simulink model "SpeedHarm"  (Simulink 8.2)
settings: Solver=ode1  StartTime=0.0  StopTime=Inf  FixedStep=0.001  RelTol=1e-3
PostLoadFcn:
  | , if any(exist('dsrtsu_mdlpostloadfcn', 'file') == [2, 3, 6]), try dsrtsu_mdlpostloadfcn('Execute', bdroot); catch fprintf('Error in PostLoadFcn (dsrtsu_mdlpostloadfcn) for model "%s":\n %s\n', bdroot, lasterr); end, end,
undefined symbols (not defined in the file): AccelCommandMode, AutoStateEnum, command_mode, max_accel_m_s2, override_enabled, speed_command_m_s, wrench_effort_command
libraries: simulink x33, carma_platform x3, srx_platform x3, dsrc_transmitter x2, rtiethernetudplib x2, rtitttasklib x2, parse_utils x1, rtican x1
(part 1 of 2)
settings Model: DSRTSU_INTERNAL_RTI_VER=450  DSRTSU_INTERNAL_RTI_TYPE=rti1401  DSRTSU_INTERNAL_RTIFPGA=40  Creator=rushk1  LastModifiedBy=leslieem  BufferReuse=off
settings DataIOCC: SignalLoggingSaveFormat=Dataset
settings OptimizationCC: BlockReduction=off  OptimizeBlockIOStorage=off  BufferReuse=off  ExpressionFolding=off  ExpressionDepthLimit=128  LocalBlockOutputs=off
settings DebuggingCC: FcnCallInpInsideContextMsg=EnableAllAsError  StateNameClashWarn=none
settings HardwareCC: ProdIntDivRoundTo=Zero  ProdEndianess=BigEndian  ProdHWDeviceType=Generic->Custom  TargetHWDeviceType=Generic->Custom
settings RTWCC: SystemTargetFile=rti1401.tlc  MakeCommand=make_rti  TemplateMakefile=rti1401.tmf  Description=dSPACE DS1401 Hardware Platform  ProcessScript=rti1401_make_rtw_hook  CustomSource=command_accel_encode.c
settings STFCustomTargetCC: CodeReplacementLibrary=ANSI_C  ParMdlRefBuildCompliant=on  GeneratePreprocessorConditionals=Disable all  SystemTargetFile=rti1401.tlc
settings GRTTargetCC: CompOptLevelCompliant=off  ConcurrentExecutionCompliant=off  MatFileLogging=off  ExtModeMexFile=noextcomm
settings CustomProperty: DataType=RTWOptions_EnumType_C__Program Files_dSPACE RCPHIL 2014-B_MATLAB_RTI_RTI1401_TLC_rti1401_1InitialSimState  Value=RUN
settings EnumStrPairs: String=RUN

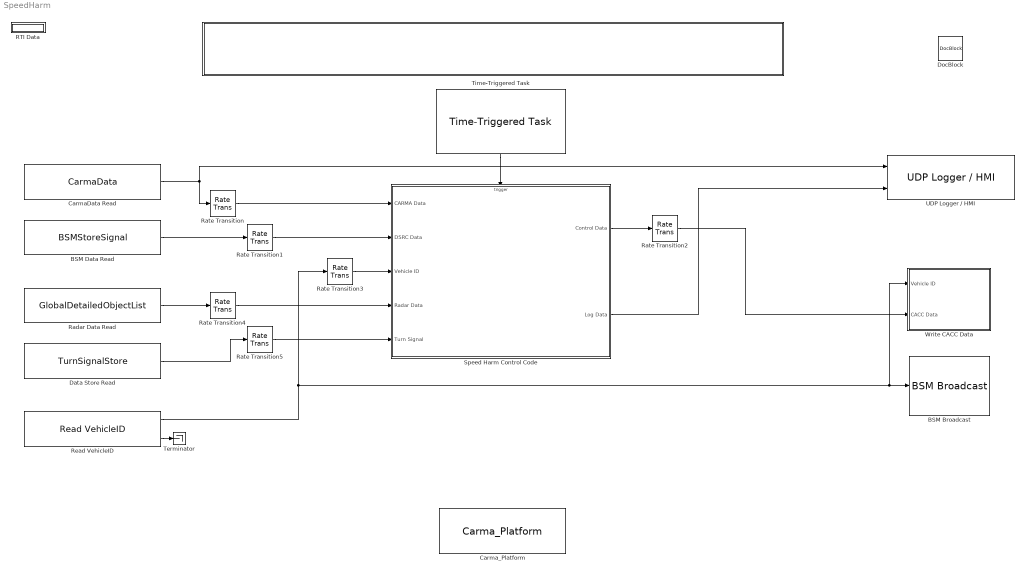
== system SpeedHarm ==
  " " : Subsystem
      mask Display: disp('Speed Harm Control Software\nTOPR 22\n2016')
  BSM Broadcast : dsrc_transmitter/BSM Broadcast
  BSM Data Read : DataStoreRead  DataStoreName=BSMStoreSignal
  CarmaData Read : DataStoreRead  DataStoreName=CarmaData
  "Carma_Platform " : carma_platform/Carma_Platform 
  Data Store Read : DataStoreRead  DataStoreName=TurnSignalStore
  DocBlock : simulink/Model-Wide Utilities/DocBlock  DocumentType=Text
  RTI Data : Subsystem  Tag=struct('RTIDataServer',struct('RTIDataServerVs','2','RTIModelDescription','struct(''main'',''SpeedHarm'',''sub'',''SpeedHarm'',''isMp'',0)'))  LoadFcn="if exist('rtidc'), try,  rtidc('DataHostBlockClbLoad', gcbh); catch, disp(['Warning: ''LoadFcn'' for RTI Data block failed: ' lasterr]); end, end,"  mask(RTI_DATA_HOST){}
      mask help:
      | RTI Data Block.
      | This block is used by RTI to store internal model-dependent data.
      | Please keep this block on the root level of the model. Deleting this block will result in data loss.
      |
      | NEVER DELETE OR COPY THIS BLOCK!
      settings: CopyFcn="if exist('rtidc'), try,  rtidc('DataHostBlockClbCopy', gcbh); catch, disp(['Warning: ''CopyFcn'' for RTI Data block failed: ' lasterr]); end, end,"  DeleteFcn="if exist('rtidc'), try,  rtidc('DataHostBlockClbDelete', gcbh); catch, disp(['Warning: ''DeleteFcn'' for RTI Data block failed: ' lasterr]); end, end,"  ModelCloseFcn="if exist('rtidc'), try,  rtidc('DataHostBlockClbModelClose', gcbh); catch, disp(['Warning: ''ModelCloseFcn'' for RTI Data block failed: ' lasterr]); end, end,"  PreSaveFcn="if exist('rtidc'), try,  rtidc('DataHostBlockClbPreSave', gcbh); catch, disp(['Warning: ''PreSaveFcn'' for RTI Data block failed: ' lasterr]); end, end,"  PostSaveFcn="if exist('rtidc'), try,  rtidc('DataHostBlockClbPostSave', gcbh); catch, disp(['Warning: ''PostSaveFcn'' for RTI Data block failed: ' lasterr]); end, end,"  NameChangeFcn="if exist('rtidc'), try,  rtidc('DataHostBlockClbNameChange', gcbh); catch, disp(['Warning: ''NameChangeFcn'' for RTI Data block failed: ' lasterr]); end, end,"
      mask Help:
      | RTI Data Block.
      | This block is used by RTI to store internal model-dependent data.
      | Please keep this block on the root level of the model. Deleting this block will result in data loss.
      | 
      | NEVER DELETE OR COPY THIS BLOCK!
      mask Display:
      | text(0.5, 0.5, 'RTI Data', 'HorizontalAlignment', 'center');
      | plot([1 0]);
  Radar Data Read : DataStoreRead  DataStoreName=GlobalDetailedObjectList
  Rate Transition{,1..5} (6 alike) : RateTransition  Deterministic=off
  Read VehicleID : srx_platform/Read VehicleID
  Speed Harm Control Code : Subsystem
  Terminator : Terminator
  Time-Triggered Task : rtitttasklib/Time-Triggered Task  TimeTriggerId=ALGO_EXEC  TLCFileName=rtitimetriggeredtask  DSProperties=struct('RTI',struct('Version',uint32(1),'BlockType',struct('isSLSource',uint8(1),'isSLSink',uint8(0),'isHWSource',uint8(0),'isHWSink',uint8(0),'isSetup',uint8(0),'isInline',uint8(1),'isNonInline',uint8(0),'isInterrupt',uint8(0),'isChannelwise',uint8(0)),'IOBoardType','RTITIMETRIGGER','UnitType','TIMETRIGGERED','Identifier','TASK','DialogType','SL','BlockSet','NONE','SlaveProcessor','NONE'))  RTIBlockInterface=struct('OutputPortsActive',1,'OutputPortsWidth',int32(1),'FunctionCall',uint32(0),'OutputPortsName',{{[' ']}},'InitLevel',3,'BlockDisplay',{{['Time-Triggered Task\nID: ''''ALGO_EXEC'''''],'center'}},'IconTransparency','off','BlockName',struct('Token',{{['Time-Triggered Task']}}),'MaskDescription',['Specifies a time-triggered task. The task trigger times are set by the assigned Time-Trigger Set block.' char(10) '' char(10) 'This block can only be used together with the Time-Trigger Set block.'])  RTIBlockParameters=struct('TimeTriggerId',{{'ALGO_EXEC','OFF',[]}},'TLCFileName',{{'rtitimetriggeredtask','OFF',[]}})  RTISFcnParameters=struct('TLCFileName','char')  RTIBlockParaDefault=struct('TimeTriggerId','TT_ID','TLCFileName','rtitimetriggeredtask')
  UDP Logger / HMI : carma_platform/UDP Logger // HMI  Value=0.05
  Write CACC Data : Subsystem  AncestorBlock=dsrc_transmitter/Write CACC Data
  wires:
  BSM Data Read/1 -> Rate Transition1/1
  CarmaData Read/1 -> Rate Transition/1, UDP Logger / HMI/1
  Rate Transition1/1 -> Speed Harm Control Code/2(DSRC Data)
  Speed Harm Control Code/2(Log Data) -> UDP Logger / HMI/2
  Speed Harm Control Code/1(Control Data) -> Rate Transition2/1
  Read VehicleID/2 -> Terminator/1
  Read VehicleID/1 -> Write CACC Data/1(Vehicle ID), BSM Broadcast/1, Rate Transition3/1
  Rate Transition2/1 -> Write CACC Data/2(CACC Data)
  Time-Triggered Task/1 -> Speed Harm Control Code/Trigger
  Rate Transition3/1 -> Speed Harm Control Code/3(Vehicle ID)
  Rate Transition/1 -> Speed Harm Control Code/1(CARMA Data)
  Radar Data Read/1 -> Rate Transition4/1
  Rate Transition4/1 -> Speed Harm Control Code/4(Radar Data)
  Data Store Read/1 -> Rate Transition5/1
  Rate Transition5/1 -> Speed Harm Control Code/5(Turn Signal)

== system SpeedHarm/  ==

== system SpeedHarm/RTI Data ==
  RTI Data Store : Subsystem  Tag=struct('private',struct('version',struct('dsVer',uint32(2)),'access',struct('modified',['03-May-2016 18:00:07'],'type','Model','isPerm',1)))  mask(RTI_DATA_STORE){}
      mask help:
      | RTI Data Store Block. This block is used by RTI to store internal model dependent data. Deleting this block will result in data loss.
      |
      | NEVER DELETE, COPY, OR MODIFY THIS BLOCK!
      mask Help:
      | RTI Data Store Block. This block is used by RTI to store internal model dependent data. Deleting this block will result in data loss.
      | 
      | NEVER DELETE, COPY, OR MODIFY THIS BLOCK!
      mask Display: text(0.5, 0.5, ' ', 'HorizontalAlignment', 'center');

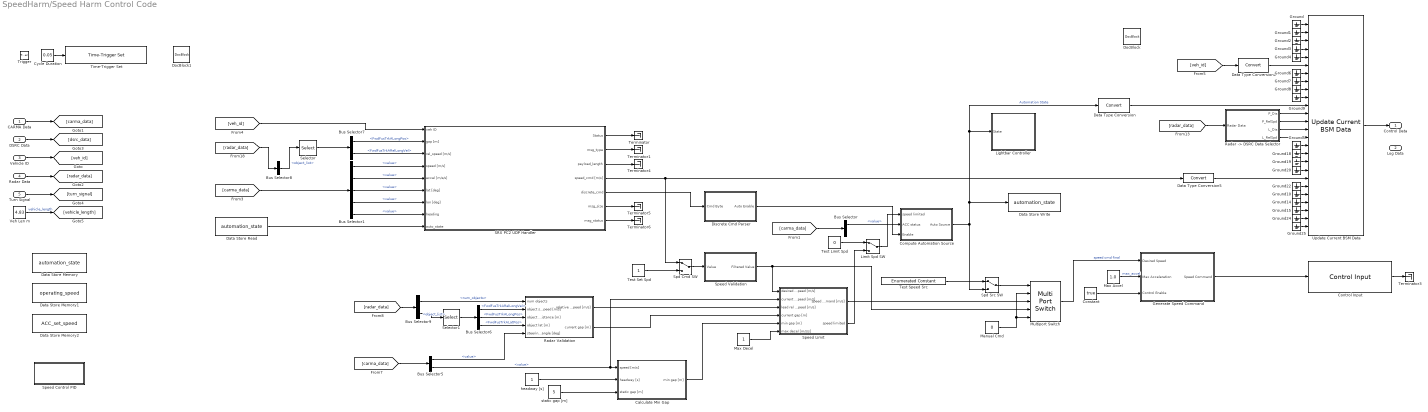
== system SpeedHarm/Speed Harm Control Code ==
  CARMA Data : Inport
  DSRC Data : Inport  Port=2
  Vehicle ID : Inport  Port=3
  Radar Data : Inport  Port=4  OutDataTypeStr=Bus: DetailedObjectList
  Turn Signal : Inport  Port=5
  Trigger : TriggerPort  TriggerType=function-call  PortDimensions=1
  Bus Selector : BusSelector  OutputSignals=acc_status.value,requested_cacc_state.value
  Bus Selector1 : BusSelector  OutputSignals=speed_m_s.value,accel_m_s2.value,global_lat_deg.value,global_long_deg.value,global_yaw_deg.value
  Bus Selector5 : BusSelector  OutputSignals=steering_wheel_angle_deg.value,speed_m_s.value
  Bus Selector6 : BusSelector  OutputSignals=FwdFusTrkARelLongVel,FwdFusTrkALongPos,FwdFusTrkALatPos
  Bus Selector7 : BusSelector  OutputSignals=FwdFusTrkALongPos,FwdFusTrkARelLongVel
  Bus Selector8 : BusSelector  OutputSignals=object_list
  Bus Selector9 : BusSelector  OutputSignals=num_objects,object_list
  Calculate Min Gap : Subsystem
  Compute Automation Source : Subsystem
  Constant : Constant  Value=true
  Control Input : carma_platform/Control Input
  Cycle Duration : Constant  Value=0.05
  Data Store Memory : DataStoreMemory  DataStoreName=automation_state  ReadBeforeWriteMsg=warning  WriteAfterWriteMsg=warning  WriteAfterReadMsg=warning  InitialValue=AutoStateEnum.MANUAL  OutDataTypeStr=Enum: AutoStateEnum
  Data Store Memory1 : DataStoreMemory  DataStoreName=operating_speed  ReadBeforeWriteMsg=warning  WriteAfterWriteMsg=warning  WriteAfterReadMsg=warning  InitialValue=25
  Data Store Memory2 : DataStoreMemory  DataStoreName=ACC_set_speed  ReadBeforeWriteMsg=warning  WriteAfterWriteMsg=warning  WriteAfterReadMsg=warning  InitialValue=25
  Data Store Read : DataStoreRead  DataStoreName=automation_state  DataStoreElements=automation_state
  Data Store Write : DataStoreWrite  DataStoreName=automation_state  DataStoreElements=automation_state
  Data Type Conversion : DataTypeConversion
  Data Type Conversion1 : DataTypeConversion
  Data Type Conversion5 : DataTypeConversion
  Discrete Cmd Parser : Subsystem
  DocBlock : simulink/Model-Wide Utilities/DocBlock  DocumentType=Text
  DocBlock1 : simulink/Model-Wide Utilities/DocBlock  DocumentType=Text
      content=|
      | Speed Harmonization Control Code
      | ===========================================================================
      | This subystem contains all of the algorithm logic for the Speed
      | Harmonization (Speed Harm) application.
      |
      | This logic is executed at a 20hz timestep with hard real time deadlines.
      | During each iteration the following steps are performed:
      |
      | 1) Receive inputs from the platform. The latest data are gathered from the
      | relevant storage buffers (being updated by other code on independent time
      | basis) and used to perform new computations.
      | 2) Receive speed command from Secondary PC
      | 3) Package vehicle data to send to Secondary PC
      | 4) Broadcast data. The new state, speed command, and other data is written
      | into the appropriate DSRC buffers and broadcasted.
  Generate Speed Command : Subsystem
  Ground{,1..10,14..15,18..20,22,24..25} (19 alike) : Ground
  Lightbar Controller : Subsystem
  Limit Spd SW : ManualSwitch
  Manual Cmd : Constant  Value=0
  Max Accel : Constant  Value=1.0
  Max Decel : Constant
  Multiport Switch : MultiPortSwitch  DataPortOrder=Specify indices  DataPortIndices={AutoStateEnum.MANUAL, AutoStateEnum.AUTO_LOCAL, AutoStateEnum.AUTO_FULL}  DataPortForDefault=Additional data port
  "Radar -> DSRC Data Selector" : Subsystem
  Radar Validation : Subsystem
  SRX PC2 UDP Handler : Subsystem
  Selector : Selector  IndexMode=Zero-based  InputPortWidth=4  IndexOptions=Index vector (dialog)  Indices=[0]  OutputSizes=1
  Selector1 : Selector  IndexMode=Zero-based  InputPortWidth=4  IndexOptions=Index vector (dialog)  Indices=[0]  OutputSizes=1
  Spd Cmd SW : ManualSwitch
  Spd Src SW : ManualSwitch
  Speed Control PID : Subsystem
  Speed Limit : Subsystem
  Speed Validation : Subsystem
  Terminator{,1,3..6} (6 alike) : Terminator
  Test Limit Spd : Constant  Value=0
  Test Set Spd : Constant
  Test Speed Src : simulink/Sources/Enumerated Constant  OutDataTypeStr=Enum: AutoStateEnum  Value=AutoStateEnum.AUTO_FULL  SampleTime=inf
  Time-Trigger Set : rtitttasklib/Time-Trigger Set  TimeTriggerId=ALGO_EXEC  SampleTime=-1  RegisterAtSimulationStart=on  TLCFileName=rtitimetriggerset  DSProperties=struct('RTI',struct('Version',uint32(1),'BlockType',struct('isSLSource',uint8(1),'isSLSink',uint8(0),'isHWSource',uint8(0),'isHWSink',uint8(0),'isSetup',uint8(0),'isInline',uint8(1),'isNonInline',uint8(0),'isInterrupt',uint8(0),'isChannelwise',uint8(0)),'IOBoardType','RTITIMETRIGGER','UnitType','TIMETRIGGERED','Identifier','SET','DialogType','SL','BlockSet','NONE','SlaveProcessor','NONE'))  RTIBlockInterface=struct('InputPortsActive',1,'InputPortsWidth',{{'DYNAMICALLY_SIZED'}},'InputPortsDataType',{{'SS_DOUBLE'}},'InputPortsName',{{['Trigger delay']}},'InitLevel',3,'BlockDisplay',{{['Time-Trigger Set\nID: ''''ALGO_EXEC'''''],'center'}},'IconTransparency','on','BlockName',struct('Token',{{['Time-Trigger Set']}}),'MaskDescription',['When this block is evaluated it sets the task trigger times for the assigned time-triggered task.' char(10) '' char(10) 'This block can only be used together with the Time-Triggered Task block.'],'SampleTime',{{-1}})  RTIBlockParameters=struct('TimeTriggerId',{{'ALGO_EXEC','OFF',[]}},'SampleTime',{{-1,'OFF',[]}},'RegisterAtSimulationStart',{{logical(1),'OFF',[]}},'TLCFileName',{{'rtitimetriggerset','OFF',[]}})  RTISFcnParameters=struct('TimeTriggerId','char','SampleTime','double','TLCFileName','char','RegisterAtSimulationStart','double')  RTIBlockParaDefault=struct('TimeTriggerId','TT_ID','SampleTime',-1,'RegisterAtSimulationStart',0,'TLCFileName','rtitimetriggerset')
  Update Current BSM Data : dsrc_transmitter/Update Current BSM Data
  Veh Len m : Constant  Value=4.83
  headway [s] : Constant
  static gap [m] : Constant  Value=5
  Control Data : Outport
  Log Data : Outport  Port=2
  wires:
  Vehicle ID/1 -> [veh_id]
  Cycle Duration/1 -> Time-Trigger Set/1
  Update Current BSM Data/1 -> Control Data/1
  Ground/1 -> Update Current BSM Data/1
  Ground1/1 -> Update Current BSM Data/2
  Ground2/1 -> Update Current BSM Data/3
  Ground3/1 -> Update Current BSM Data/4
  Ground4/1 -> Update Current BSM Data/5
  Ground9/1 -> Update Current BSM Data/10
  Ground7/1 -> Update Current BSM Data/8
  Ground8/1 -> Update Current BSM Data/9
  Ground6/1 -> Update Current BSM Data/7
  Ground22/1 -> Update Current BSM Data/21
  Ground15/1 -> Update Current BSM Data/24
  Ground19/1 -> Update Current BSM Data/18
  Ground18/1 -> Update Current BSM Data/17
  Ground14/1 -> Update Current BSM Data/23
  Ground20/1 -> Update Current BSM Data/19
  Ground24/1 -> Update Current BSM Data/25
  Ground25/1 -> Update Current BSM Data/26
  Radar Data/1 -> [radar_data]
  CARMA Data/1 -> [carma_data]
  Compute Automation Source/1(Auto Source) -> Data Type Conversion/1, Lightbar Controller/1(State), Data Store Write/1, Spd Src SW/2  "Automation State"
  Data Type Conversion1/1 -> Update Current BSM Data/6
  [carma_data] -> Bus Selector/1
  DSRC Data/1 -> [dsrc_data]
  [veh_id] -> Data Type Conversion1/1
  Ground10/1 -> Update Current BSM Data/22
  SRX PC2 UDP Handler/1(Status) -> Terminator/1
  Control Input/1 -> Terminator3/1
  Speed Validation/1(Filtered Value) -> Multiport Switch/4, Speed Limit/1(desired speed [m/s])
  Generate Speed Command/1(Speed Command) -> Control Input/1
  Max Accel/1 -> Generate Speed Command/2(Max Acceleration)  "max_accel"
  Turn Signal/1 -> [turn_signal]
  Ground5/1 -> Update Current BSM Data/16
  [radar_data] -> "Radar -> DSRC Data Selector"/1(Radar Data)
  "Radar -> DSRC Data Selector"/1(P_Dis) -> Update Current BSM Data/12
  "Radar -> DSRC Data Selector"/2(P_RelSpd) -> Update Current BSM Data/13
  "Radar -> DSRC Data Selector"/3(L_Dis) -> Update Current BSM Data/14
  "Radar -> DSRC Data Selector"/4(L_RelSpd) -> Update Current BSM Data/15
  Data Type Conversion5/1 -> Update Current BSM Data/20
  Veh Len m/1 -> [vehicle_length]  "vehicle_length"
  static gap [m]/1 -> Calculate Min Gap/3(static gap [m])
  SRX PC2 UDP Handler/6(msg_size) -> Terminator5/1
  Bus Selector7/1 -> SRX PC2 UDP Handler/2(gap [m])  "<FwdFusTrkALongPos>"
  [carma_data] -> Bus Selector1/1
  Bus Selector1/1 -> SRX PC2 UDP Handler/4(speed [m/s])  "<value>"
  Bus Selector1/2 -> SRX PC2 UDP Handler/5(accel [m/s/s])  "<value>"
  Bus Selector1/3 -> SRX PC2 UDP Handler/6(lat [deg])  "<value>"
  Bus Selector1/4 -> SRX PC2 UDP Handler/7(lon [deg])  "<value>"
  SRX PC2 UDP Handler/7(msg_status) -> Terminator6/1
  SRX PC2 UDP Handler/3(payload_length) -> Terminator4/1
  SRX PC2 UDP Handler/2(msg_type) -> Terminator1/1
  [veh_id] -> SRX PC2 UDP Handler/1(veh ID)
  Bus Selector1/5 -> SRX PC2 UDP Handler/8(heading)  "<value>"
  Bus Selector7/2 -> SRX PC2 UDP Handler/3(rel_speed [m/s])  "<FwdFusTrkARelLongVel>"
  SRX PC2 UDP Handler/4(speed_cmd [m/s]) -> Spd Cmd SW/1, Data Type Conversion5/1
  Constant/1 -> Generate Speed Command/3(Control Enable)
  headway [s]/1 -> Calculate Min Gap/2(headway [s])
  [carma_data] -> Bus Selector5/1
  Bus Selector5/2 -> Speed Limit/2(current speed [m/s]), Calculate Min Gap/1(speed [m/s])  "<value>"
  Bus Selector6/2 -> Radar Validation/3(object distance [m])  "<FwdFusTrkALongPos>"
  Calculate Min Gap/1(min gap [m]) -> Speed Limit/5(min gap [m])
  Radar Validation/2(current gap [m]) -> Speed Limit/4(current gap [m])
  Bus Selector9/1 -> Radar Validation/1(num objects)  "<num_objects>"
  Radar Validation/1(relative speed [m/s]) -> Speed Limit/3(lead rel speed [m/s])
  Bus Selector6/1 -> Radar Validation/2(object speed [m/s])  "<FwdFusTrkARelLongVel>"
  Speed Limit/1(speed command [m/s]) -> Multiport Switch/3
  [radar_data] -> Bus Selector8/1
  Bus Selector8/1 -> Selector/1  "<object_list>"
  Selector/1 -> Bus Selector7/1
  Selector1/1 -> Bus Selector6/1
  Bus Selector9/2 -> Selector1/1  "<object_list>"
  Data Type Conversion/1 -> Update Current BSM Data/11
  SRX PC2 UDP Handler/5(discrete_cmd) -> Discrete Cmd Parser/1(Cmd Byte)
  Data Store Read/1 -> SRX PC2 UDP Handler/9(auto_state)
  Manual Cmd/1 -> Multiport Switch/5, Multiport Switch/2
  [radar_data] -> Bus Selector9/1
  Discrete Cmd Parser/1(Auto Enable) -> Compute Automation Source/3(Enable)
  Limit Spd SW/1 -> Compute Automation Source/1(speed limited)
  Test Set Spd/1 -> Spd Cmd SW/2
  Spd Cmd SW/1 -> Speed Validation/1(Value)
  Multiport Switch/1 -> Generate Speed Command/1(Desired Speed)  "speed cmd final"
  Test Speed Src/1 -> Spd Src SW/1
  Spd Src SW/1 -> Multiport Switch/1
  Bus Selector/1 -> Compute Automation Source/2(ACC status)  "<value>"
  Test Limit Spd/1 -> Limit Spd SW/1
  Max Decel/1 -> Speed Limit/6(max decel [m/s/s])
  Speed Limit/2(speed limited) -> Limit Spd SW/2
  Bus Selector5/1 -> Radar Validation/5(steering angle [deg])  "<value>"
  Bus Selector6/3 -> Radar Validation/4(object lat [m])  "<FwdFusTrkALatPos>"

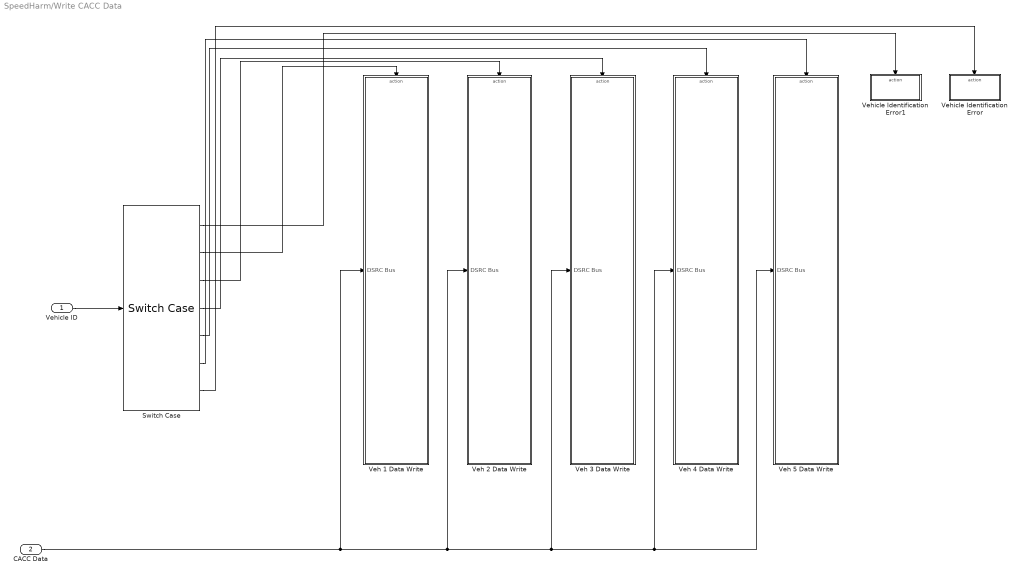
== system SpeedHarm/Write CACC Data ==
  Vehicle ID : Inport
  CACC Data : Inport  Port=2
  Switch Case : SwitchCase  CaseConditions={0,96,97,98,99,100}
  Veh 1 Data Write : Subsystem  TreatAsAtomicUnit=on
  Veh 2 Data Write : Subsystem  TreatAsAtomicUnit=on
  Veh 3 Data Write : Subsystem  TreatAsAtomicUnit=on
  Veh 4 Data Write : Subsystem  TreatAsAtomicUnit=on
  Veh 5 Data Write : Subsystem  TreatAsAtomicUnit=on
  Vehicle Identification Error : Subsystem  TreatAsAtomicUnit=on
  Vehicle Identification Error1 : Subsystem  TreatAsAtomicUnit=on
  wires:
  Vehicle ID/1 -> Switch Case/1
  Switch Case/7 -> Vehicle Identification Error/Action
  Switch Case/1 -> Vehicle Identification Error1/Action
  Switch Case/6 -> Veh 5 Data Write/Action
  Switch Case/5 -> Veh 4 Data Write/Action
  Switch Case/4 -> Veh 3 Data Write/Action
  Switch Case/3 -> Veh 2 Data Write/Action
  Switch Case/2 -> Veh 1 Data Write/Action
  CACC Data/1 -> Veh 1 Data Write/1(DSRC Bus), Veh 2 Data Write/1(DSRC Bus), Veh 3 Data Write/1(DSRC Bus), Veh 4 Data Write/1(DSRC Bus), Veh 5 Data Write/1(DSRC Bus)

== system SpeedHarm/RTI Data/RTI Data Store ==
  RTI Data Store : Subsystem  mask(RTI_DATA_STORE){}
      mask help:
      | RTI Data Store Block. This block is used by RTI to store internal model dependent data. Deleting this block will result in data loss.
      |
      | NEVER DELETE, COPY, OR MODIFY THIS BLOCK!
      mask Help:
      | RTI Data Store Block. This block is used by RTI to store internal model dependent data. Deleting this block will result in data loss.
      | 
      | NEVER DELETE, COPY, OR MODIFY THIS BLOCK!
      mask Display: text(0.5, 0.5, ' ', 'HorizontalAlignment', 'center');

== system SpeedHarm/Speed Harm Control Code/Calculate Min Gap ==
  speed [m/s] : Inport
  headway [s] : Inport  Port=2
  static gap [m] : Inport  Port=3
  Add : Sum
  DocBlock : simulink/Model-Wide Utilities/DocBlock  DocumentType=Text
  Product : Product
  min gap [m] : Outport
  wires:
  static gap [m]/1 -> Add/2
  speed [m/s]/1 -> Product/1
  headway [s]/1 -> Product/2
  Product/1 -> Add/1
  Add/1 -> min gap [m]/1

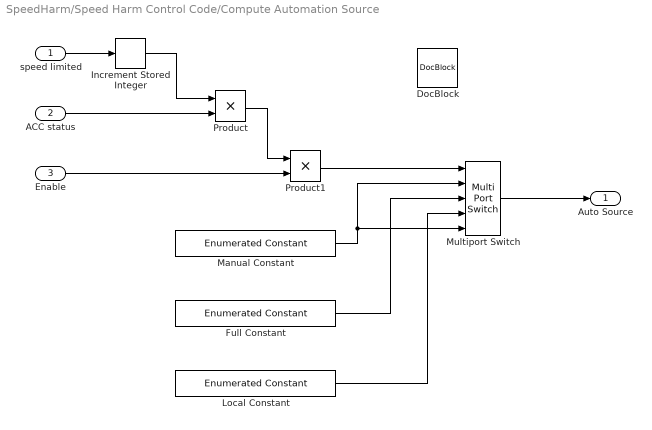
== system SpeedHarm/Speed Harm Control Code/Compute Automation Source ==
  speed limited : Inport
  ACC status : Inport  Port=2
  Enable : Inport  Port=3
  DocBlock : simulink/Model-Wide Utilities/DocBlock  DocumentType=Text
  Full Constant : simulink/Sources/Enumerated Constant  OutDataTypeStr=Enum: AutoStateEnum  Value=AutoStateEnum.AUTO_FULL  SampleTime=inf
  Increment Stored Integer : simulink/Additional Math & Discrete/Additional Math: Increment - Decrement/Increment Stored Integer
  Local Constant : simulink/Sources/Enumerated Constant  OutDataTypeStr=Enum: AutoStateEnum  Value=AutoStateEnum.AUTO_LOCAL  SampleTime=inf
  Manual Constant : simulink/Sources/Enumerated Constant  OutDataTypeStr=Enum: AutoStateEnum  Value=AutoStateEnum.MANUAL  SampleTime=inf
  Multiport Switch : MultiPortSwitch  DataPortOrder=Zero-based contiguous  DataPortForDefault=Additional data port
  Product : Product
  Product1 : Product
  Auto Source : Outport
  wires:
  Multiport Switch/1 -> Auto Source/1
  Manual Constant/1 -> Multiport Switch/5, Multiport Switch/2
  Full Constant/1 -> Multiport Switch/3
  Local Constant/1 -> Multiport Switch/4
  Product1/1 -> Multiport Switch/1
  ACC status/1 -> Product/2
  speed limited/1 -> Increment Stored Integer/1
  Increment Stored Integer/1 -> Product/1
  Product/1 -> Product1/1
  Enable/1 -> Product1/2

== system SpeedHarm/Speed Harm Control Code/Discrete Cmd Parser ==
  Cmd Byte : Inport
  Bitwise Operator : simulink/Logic and Bit Operations/Bitwise Operator  logicop=AND  UseBitMask=on  BitMask=bin2dec('00000001')  BitMaskRealWorld=Stored Integer
  DocBlock : simulink/Model-Wide Utilities/DocBlock  DocumentType=Text
  Auto Enable : Outport
  wires:
  Cmd Byte/1 -> Bitwise Operator/1
  Bitwise Operator/1 -> Auto Enable/1

== system SpeedHarm/Speed Harm Control Code/Generate Speed Command ==
  Desired Speed : Inport
  Max Acceleration : Inport  Port=2
  Control Enable : Inport  Port=3
  Accel Zero Command : Constant  Value=0  OutDataTypeStr=Bus: AccelCommandBus
  Bus Assignment : BusAssignment  AssignedSignals=override_enabled,command_mode,wrench_effort_command,speed_command_m_s,max_accel_m_s2
  Constant : Constant  Value=AccelCommandMode.SpeedControl  OutDataTypeStr=Enum: AccelCommandMode
  Constant1 : Constant  Value=0
  DocBlock : simulink/Model-Wide Utilities/DocBlock  DocumentType=Text
  Speed Command : Outport
  wires:
  Control Enable/1 -> Bus Assignment/2
  Constant1/1 -> Bus Assignment/4
  Desired Speed/1 -> Bus Assignment/5
  Max Acceleration/1 -> Bus Assignment/6
  Accel Zero Command/1 -> Bus Assignment/1
  Bus Assignment/1 -> Speed Command/1
  Constant/1 -> Bus Assignment/3

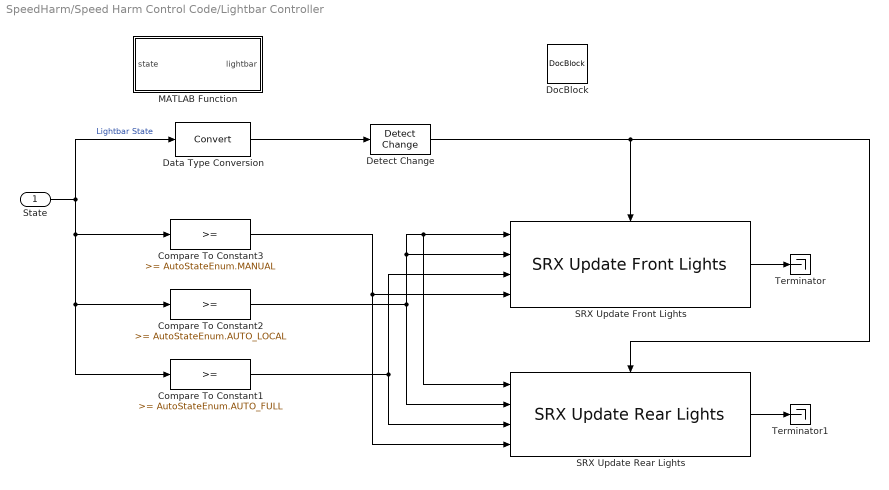
== system SpeedHarm/Speed Harm Control Code/Lightbar Controller ==
  State : Inport
  Compare To Constant1 : simulink/Logic and Bit Operations/Compare To Constant  relop=>=  const=AutoStateEnum.AUTO_FULL  OutDataTypeStr=boolean
  Compare To Constant2 : simulink/Logic and Bit Operations/Compare To Constant  relop=>=  const=AutoStateEnum.AUTO_LOCAL  OutDataTypeStr=boolean
  Compare To Constant3 : simulink/Logic and Bit Operations/Compare To Constant  relop=>=  const=AutoStateEnum.MANUAL  OutDataTypeStr=boolean
  Data Type Conversion : DataTypeConversion
  Detect Change : simulink/Logic and Bit Operations/Detect Change  vinit=0  InputProcessing=Inherited  OutDataTypeStr=boolean
  DocBlock : simulink/Model-Wide Utilities/DocBlock  DocumentType=Text
      content=|
      | This block is responsible for controlling the state of the vehicle's
      | lightbar.
      |
      | The lightbar state is dependant on the vehicle's merge state. Merge request
      | triggers the right side of the lightbar to flash. Merge request ack
      | triggers the left side of the bar to flash. Merge ready causes both sides
      | of the lightbar to flash. Once merge completion is attained the green light
      | in the center of light bar will light up solid.
  MATLAB Function : MATLAB Function  TreatAsAtomicUnit=on
  SRX Update Front Lights : srx_platform/SRX Update Front Lights
  SRX Update Rear Lights : srx_platform/SRX Update Rear Lights
  Terminator : Terminator
  Terminator1 : Terminator
  wires:
  Compare To Constant2/1 -> SRX Update Rear Lights/1, SRX Update Front Lights/1, SRX Update Front Lights/2, SRX Update Rear Lights/2
  Compare To Constant1/1 -> SRX Update Front Lights/3, SRX Update Rear Lights/3
  Compare To Constant3/1 -> SRX Update Rear Lights/4, SRX Update Front Lights/4
  Detect Change/1 -> SRX Update Front Lights/Enable, SRX Update Rear Lights/Enable
  SRX Update Front Lights/1 -> Terminator/1
  SRX Update Rear Lights/1 -> Terminator1/1
  State/1 -> Compare To Constant2/1, Compare To Constant1/1, Compare To Constant3/1, Data Type Conversion/1  "Lightbar State"
  Data Type Conversion/1 -> Detect Change/1

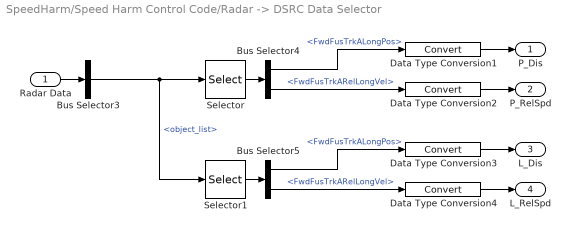
== system SpeedHarm/Speed Harm Control Code/Radar -> DSRC Data Selector ==
  Radar Data : Inport
  Bus Selector3 : BusSelector  OutputSignals=object_list
  Bus Selector4 : BusSelector  OutputSignals=FwdFusTrkALongPos,FwdFusTrkARelLongVel
  Bus Selector5 : BusSelector  OutputSignals=FwdFusTrkALongPos,FwdFusTrkARelLongVel
  Data Type Conversion{1..4} (4 alike) : DataTypeConversion
  Selector : Selector  InputPortWidth=4  IndexOptions=Index vector (dialog)  Indices=[1]  OutputSizes=1
  Selector1 : Selector  InputPortWidth=4  IndexOptions=Index vector (dialog)  Indices=[2]  OutputSizes=1
  P_Dis : Outport
  P_RelSpd : Outport  Port=2
  L_Dis : Outport  Port=3
  L_RelSpd : Outport  Port=4
  wires:
  Bus Selector5/2 -> Data Type Conversion4/1  "<FwdFusTrkARelLongVel>"
  Bus Selector5/1 -> Data Type Conversion3/1  "<FwdFusTrkALongPos>"
  Radar Data/1 -> Bus Selector3/1
  Bus Selector4/2 -> Data Type Conversion2/1  "<FwdFusTrkARelLongVel>"
  Bus Selector3/1 -> Selector1/1, Selector/1  "<object_list>"
  Bus Selector4/1 -> Data Type Conversion1/1  "<FwdFusTrkALongPos>"
  Selector1/1 -> Bus Selector5/1
  Selector/1 -> Bus Selector4/1
  Data Type Conversion1/1 -> P_Dis/1
  Data Type Conversion2/1 -> P_RelSpd/1
  Data Type Conversion3/1 -> L_Dis/1
  Data Type Conversion4/1 -> L_RelSpd/1

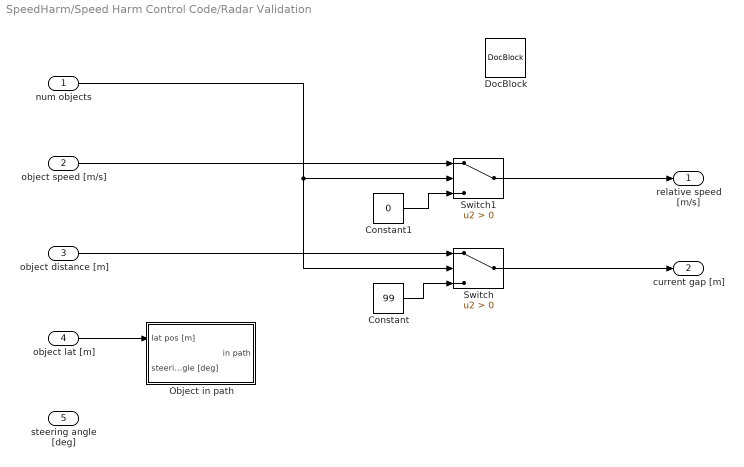
== system SpeedHarm/Speed Harm Control Code/Radar Validation ==
  num objects : Inport
  object speed [m/s] : Inport  Port=2
  object distance [m] : Inport  Port=3
  object lat [m] : Inport  Port=4
  steering angle [deg] : Inport  Port=5
  Constant : Constant  Value=99
  Constant1 : Constant  Value=0
  DocBlock : simulink/Model-Wide Utilities/DocBlock  DocumentType=Text
      content=|
      | This block outputs the radar distance and speed to the nearest object,
      | or outputs a known value if no objects are detected.
      |
      | Future work:
      | Use the radar azimuth, steering wheel angle, and other data to filter out
      | objects not in the path of this vehicle
  Object in path : Subsystem
  Switch : Switch  Criteria=u2 > Threshold
  Switch1 : Switch  Criteria=u2 > Threshold
  relative speed [m/s] : Outport
  current gap [m] : Outport  Port=2
  wires:
  num objects/1 -> Switch/2, Switch1/2
  object distance [m]/1 -> Switch/1
  Constant/1 -> Switch/3
  Switch/1 -> current gap [m]/1
  object speed [m/s]/1 -> Switch1/1
  Constant1/1 -> Switch1/3
  Switch1/1 -> relative speed [m/s]/1
  object lat [m]/1 -> Object in path/1(lat pos [m])

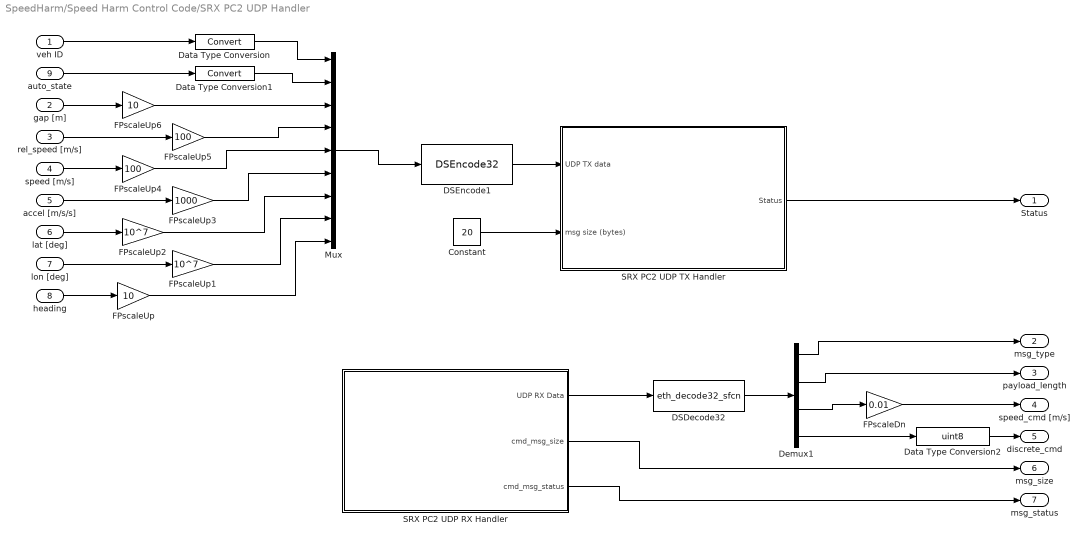
== system SpeedHarm/Speed Harm Control Code/SRX PC2 UDP Handler ==
  veh ID : Inport
  gap [m] : Inport  Port=2
  rel_speed [m/s] : Inport  Port=3
  speed [m/s] : Inport  Port=4
  accel [m/s/s] : Inport  Port=5
  lat [deg] : Inport  Port=6
  lon [deg] : Inport  Port=7
  heading : Inport  Port=8
  auto_state : Inport  Port=9
  Constant : Constant  Value=20  OutDataTypeStr=int32
  "DSDecode32 " : S-Function  FunctionName=eth_decode32_sfcn  Parameters=byteordering,offset,auto_offset,datatype,one_datatype,sampletime  EnableBusSupport=off  mask(DSDecode32){byteordering=little endian (Intel), offset=[0], auto_offset=on, datatype=[3 3 5 3], one_datatype=off, sampletime=-1}
      mask prompts: byteordering "Byte ordering:"; offset "Offset (bytes):"; auto_offset "Auto offset"; one_datatype "One datatype only"
      mask help:
      | Converts a 32bit WORD input data stream into the specified datatypes on the output port.
      |
      | Datatype Codes:
      | BOOLEAN:  1   //   INT8      :  2    //   UINT8    :  3
      | INT16       :  4   //   UINT16 :  5    //   INT32     :  6
      | UINT32    :  7   //   FLOAT   :  8    //   DOUBLE:  9
      mask Help:
      | The 'DSDecode32' block allows to decode an UInt32 vector containing encoded elements of various data types to an output vector of double values. It is intended to use this block in conjunction with the 'DS4504_ETH_Receive' block which delivers this format as data output. Data received from the Ethernet via the 'DS4504_ETH_Receive' block is performed in Intel byte order ('Little Endian').
      | 
      | <br>
      | <br>
      | 
      | <h2>Parameters</h2>
      | <br>
      | <br>
      | 
      | <b>Byte ordering (only relevant for offline simulation)</b>
      | <br>
      | <blockquote>
      | The byte order of the input vector has to be specified. In case of running a real-time application the appropriate byte order (Motorola for DS1005 and Intel for DS1006) is selected automatically. Therefore the byte order setting has no influence on the online simulation.
      | </blockquote>
      | <br>
      | 
      | <b>Offset (bytes)</b>
      | <br>
      | <blockquote>
      | This is for defining a vector of offsets which specifies the position of each element within the input vector. The offsets must be entered as an array (e.g. [1 10 . 50 54] ) using the same order as for the corresponding data type vector (see (4)). This option is useful if you have gaps between adjacent elements.
      | </blockquote>
      | <br>
      | 
      | <b>Auto offset</b>
      | <br>
      | <blockquote>
      | When activating this checkbox parameter, the edit field 'Offset' is disabled and the byte offsets in the input vector are calculated automatically concerning the specified data types (no gaps presupposed). Any previous setting in the offset vector would be ignored.
      | </blockquote>
      | <br>
      | 
      | <b>Datatype</b>
      | <br>
      | <blockquote>
      | This is for defining a vector of data types which specifies the type for each element in the input vector. Supported data types are Boolean, Int8, UInt8, Int16, UInt16, Int32, UInt32, Float and Double, which are determined by using the corresponding data type codes shown in the following table:
      | <br>
      | <br>
      | <table BORDER=1 ALIGN="center">
      | <TR>
      | <TH WIDTH=20%>Data type</TH>
      | <TH WIDTH=20%>Data type code</TH>
      | <TH WIDTH=20%>Length in bytes</TH>
      | </TR>
      | <TR><TD>Boolean</TD><TD ALIGN="center">1</TD><TD ALIGN="center">1</TD></TR>
      | <TR><TD>Int8</TD><TD ALIGN="center">2</TD><TD ALIGN="center">1</TD></TR>
      | <TR><TD>Uint8</TD><TD ALIGN="center">3</TD><TD ALIGN="center">1</TD></TR>
      | <TR><TD>Int16</TD><TD ALIGN="center">4</TD><TD ALIGN="center">2</TD></TR>
      | <TR><TD>Uint16</TD><TD ALIGN="center">5</TD><TD ALIGN="center">2</TD></TR>
      | <TR><TD>Int32</TD><TD ALIGN="center">6</TD><TD ALIGN="center">4</TD></TR>
      | <TR><TD>Uint32</TD><TD ALIGN="center">7</TD><TD ALIGN="center">4</TD></TR>
      | <TR><TD>Float</TD><TD ALIGN="center">8</TD><TD ALIGN="center">4</TD></TR>
      | <TR><TD>Double</TD><TD ALIGN="center">9</TD><TD ALIGN="center">8</TD></TR>
      | </TABLE>
      | </blockquote>
      | <br>
      | 
      | <b>One datatype only</b>
      | <br>
      | <blockquote>
      | This option is useful if all elements of the input vector have the same data type. If the checkbox is activated the first element of the data type vector specifies the data type to be used. In this case it is naturally sufficient to enter only one number which applies for the complete input vector.
      | </blockquote>
      | <br>
      | 
      | <b>Sample time</b>
      | <br>
      | <blockquote>
      | The desired sample time for this block has to be entered here. Alternatively it can be  inherited from the Simulink model by using '-1'.
      | </blockquote>
      | <br>
      mask TypeOptions byteordering: big endian (Motorola) | little endian (Intel)
      mask Display: text(0.5,0.5,'DSDecode32','HorizontalAlignment','center')
  DSEncode1 : parse_utils/DSEncode32  byteordering=little endian (Intel)  offset=[ 0 ]  auto_offset=on  datatype=[3 3 5 4 5 4 6 6 4]  one_datatype=off  sampletime=-1
  Data Type Conversion : DataTypeConversion
  Data Type Conversion1 : DataTypeConversion
  Data Type Conversion2 : DataTypeConversion  OutDataTypeStr=uint8
  Demux1 : Demux
  FPscaleDn : Gain  Gain=0.01
  FPscaleUp : Gain  Gain=10  OutDataTypeStr=double
  FPscaleUp1 : Gain  Gain=10^7
  FPscaleUp2 : Gain  Gain=10^7
  FPscaleUp3 : Gain  Gain=1000  OutDataTypeStr=double
  FPscaleUp4 : Gain  Gain=100  OutDataTypeStr=double
  FPscaleUp5 : Gain  Gain=100
  FPscaleUp6 : Gain  Gain=10
  Mux : Mux  Inputs=9
  SRX PC2 UDP RX Handler : Subsystem
  SRX PC2 UDP TX Handler : Subsystem
  Status : Outport
  msg_type : Outport  Port=2
  payload_length : Outport  Port=3
  speed_cmd [m/s] : Outport  Port=4
  discrete_cmd : Outport  Port=5
  msg_size : Outport  Port=6
  msg_status : Outport  Port=7
  wires:
  SRX PC2 UDP RX Handler/2(cmd_msg_size) -> msg_size/1
  SRX PC2 UDP RX Handler/3(cmd_msg_status) -> msg_status/1
  SRX PC2 UDP TX Handler/1(Status) -> Status/1
  Mux/1 -> DSEncode1/1
  gap [m]/1 -> FPscaleUp6/1
  heading/1 -> FPscaleUp/1
  lon [deg]/1 -> FPscaleUp1/1
  lat [deg]/1 -> FPscaleUp2/1
  accel [m/s/s]/1 -> FPscaleUp3/1
  speed [m/s]/1 -> FPscaleUp4/1
  rel_speed [m/s]/1 -> FPscaleUp5/1
  SRX PC2 UDP RX Handler/1(UDP RX Data) -> "DSDecode32 "/1
  Demux1/1 -> msg_type/1
  Demux1/2 -> payload_length/1
  DSEncode1/1 -> SRX PC2 UDP TX Handler/1(UDP TX data)
  "DSDecode32 "/1 -> Demux1/1
  Demux1/3 -> FPscaleDn/1
  Demux1/4 -> Data Type Conversion2/1
  FPscaleDn/1 -> speed_cmd [m/s]/1
  FPscaleUp/1 -> Mux/9
  FPscaleUp1/1 -> Mux/8
  FPscaleUp2/1 -> Mux/7
  FPscaleUp3/1 -> Mux/6
  FPscaleUp4/1 -> Mux/5
  FPscaleUp5/1 -> Mux/4
  FPscaleUp6/1 -> Mux/3
  veh ID/1 -> Data Type Conversion/1
  auto_state/1 -> Data Type Conversion1/1
  Constant/1 -> SRX PC2 UDP TX Handler/2(msg size (bytes))
  Data Type Conversion1/1 -> Mux/2
  Data Type Conversion/1 -> Mux/1
  Data Type Conversion2/1 -> discrete_cmd/1

== system SpeedHarm/Speed Harm Control Code/Speed Control PID ==
  DocBlock : simulink/Model-Wide Utilities/DocBlock  DocumentType=Text
      content=|
      | The Ohio State University - Lane Change/Merge Vehicle Testing - TOPR20
      |
      | Researcher CAN speed controller PID values (check the excel sheet for hex information)
  Speed Control PID Parameters : rtican/RTICAN Receive (RX)   Reserved1=[]  Reserved2=[]  Reserved3=[]  Reserved4=[]  SfcnMessage=[]  Msg_Struct=[]  BoardTypeNo=[]  BoardNo=[]  ChannelNo=[]  Parameters=[]  DialogFcn=[]  UnitName=[]  Revision=[]  UnitValues=[]  DSProperties=struct('RTI',struct('Version',uint32(5),'BlockType',struct('isSLSource',uint8(1),'isSLSink',uint8(1),'isHWSource',uint8(0),'isHWSink',uint8(0),'isSetup',uint8(0),'isInline',uint8(1),'isNonInline',uint8(0),'isInterrupt',uint8(0),'isChannelwise',uint8(0)),'IOBoardType','RTICAN','UnitType','MESSAGE','Identifier','RX','DialogType','MSVC','BlockSet','RTICAN','SlaveProcessor','CAN'))  RTIBlockInterface=struct('OutputPortsWidth',int32([1 1 1 1 1 1 1]),'OutputPortsActive',[1 1 1 1 1 1 1],'OutputPortsName',{{'PGainNumerator','IGainNumerator','DGainNumerator','PIDDivisor',['RX status'],['RX time'],['RX delta time']}},'OutputPortsDataType',{{'SS_UINT16','SS_UINT16','SS_UINT16','SS_UINT16','SS_DOUBLE','SS_DOUBLE','SS_DOUBLE'}},'OutputPortsLabel',{{'PGainNumerator','IGainNumerator','DGainNumerator','PIDDivisor','','',''}},'OutputPortsLabelMode','ON','InputPortsWidth',int32(0),'InputPortsActive',0,'DialogFcn','rtican_message_interface_gui','BlockDisplay',{{'','center'}},'IconTransparency','on','ParameterTunableNames',{{}},'InitLevel',3,'BlockName',struct('Token',{{'CAN_TYPE','_RX_M','_C'}},'BlockParam',{{'BoardTypeNo','BoardNo','ChannelNo'}}),'SampleTime',{{-1}},'TriggerPort',{{'none'}},'EnablePort',{{'none'}})  RTIBlockParameters=struct('BoardTypeNo',{{1,'OFF',[]}},'BoardNo',{{2,'ON',[1 16]}},'ChannelNo',{{1,'ON',[1 2]}},'Parameters',{{struct('DataFileSupport',struct('DataFileSelectedMaster',1,'DataFileSelectedLocal',0,'DataFileName',['c:\users\leslieem\documents\topr 22\control\speedharm22-mab\src\data_files\srx_command.dbc|'],'DataFileDate','','SelectedFile',['<no file selected>']),'Options',struct('StatusSelected',1,'TimeSelected',1,'DeltaTimeSelected',1,'BytePortSelected',0,'MessageLengthSelected',0,'TriggerPort',struct('Selected',0,'TriggerType',0),'UserCoding',struct('Selected',0,'InterfaceFile','UserDecodingFile','FcnName','UserDecodeFcn','InportSelected',0,'InportWidth',1,'OutportSelected',0,'OutportWidth',1),'EnablePortSelected',0,'SignalOnPortnameSelected',1,'UseRXService',0),'Message',struct('MsgOnBlocknameSelected',0,'MsgName',['RX Message'],'MsgIdFormat',0,'MsgId',273,'MsgLength',8,'NumSignals',4,'SampleTime',-1,'Signal',struct('SgnName',{'PGainNumerator','IGainNumerator','DGainNumerator','PIDDivisor'},'SgnStartBit',{0,16,32,48},'SgnLength',{16,16,16,16},'SgnType',{0,0,0,0},'ModeValue',{-1,-1,-1,-1},'DataType',{0,0,0,0},'ByteLayout',{1,1,1,1},'Factor',{1,1,1,1},'Offset',{0,0,0,0},'SgnComment',{{''},{''},{''},{''}},'SgnUnit',{'','','',''},'Min',{0,0,0,0},'Max',{255,255,255,255},'SLDataType',{'SS_UINT16','SS_UINT16','SS_UINT16','SS_UINT16'}),'MsgIdNumFormat',1,'MsgComment',{{''}}),'Version',1.2,'general',struct('isFromLib',0)),'OFF',[]}},'GroupId',{{struct('Group',{{'RTICAN'}},'No',3,'Behavior',{{'NAMECHANGE'}},'BlockType',{{'SINK'}},'NameChangeFlag',0),'OFF',[]}},'SFcnRTICANMessage',{{struct('MsgType','RX','SFcnPortType','Scalar','MsgName',['RX Message'],'MsgIdFormat','STD','MsgId',273,'MsgLength',8,'NumSignals',4,'SampleTime',-1,'Signal',struct('SgnName',{'PGainNumerator','IGainNumerator','DGainNumerator','PIDDivisor'},'SgnStartBit',{0,16,32,48},'SgnLength',{16,16,16,16},'SgnType',{'standard','standard','standard','standard'},'ModeValue',{-1,-1,-1,-1},'DataType',{['unsigned int'],['unsigned int'],['unsigned int'],['unsigned int']},'ByteLayout',{['big endian'],['big endian'],['big endian'],['big endian']},'Factor',{1,1,1,1},'Offset',{0,0,0,0},'SLDataType',{'SS_UINT16','SS_UINT16','SS_UINT16','SS_UINT16'}),'StatusSelected','yes','TimeSelected','yes','DeltaTimeSelected','yes','BytePortSelected','no','MessageLengthSelected','no','TriggerPort',struct('Selected','no','TriggerType',0),'UserCoding',struct('Selected','no','InterfaceFile','UserDecodingFile','FcnName','UserDecodeFcn','InportSelected','no','InportWidth',1,'OutportSelected','no','OutportWidth',1),'EnablePortSelected','no','UseRXService','no','BoardType','DS1','BoardNo',1,'ControllerNo',1),'OFF',[]}},'TLCFileName',{{'rtican_rx_message','OFF',[]}})  RTISFcnParameters=struct('SFcnRTICANMessage','struct','TLCFileName','char')  RTIBlockParaDefault=struct('BoardTypeNo',4302,'BoardNo',1,'ChannelNo',1,'Parameters',struct('DataFileSupport',struct('DataFileSelectedMaster',0,'DataFileSelectedLocal',0,'DataFileName','','DataFileDate','','SelectedFile',['<no file selected>']),'Options',struct('StatusSelected',1,'TimeSelected',1,'DeltaTimeSelected',1,'BytePortSelected',0,'MessageLengthSelected',0,'TriggerPort',struct('Selected',0,'TriggerType','rising'),'UserCoding',struct('Selected',0,'InterfaceFile','UserDecodingFile','FcnName','UserDecodeFcn','InportSelected',0,'InportWidth',1,'OutportSelected',0,'OutportWidth',1),'EnablePortSelected',0,'SignalOnPortnameSelected',1,'UseRXService',0),'Message',struct('MsgOnBlocknameSelected',0,'MsgName',['RX Message'],'MsgIdFormat',0,'MsgId',100,'MsgLength',8,'NumSignals',1,'SampleTime',-1,'Signal',struct('SgnName',['RX signal'],'SgnStartBit',0,'SgnLength',8,'SgnType',0,'ModeValue',-1,'DataType',0,'SLDataType','SS_DOUBLE','ByteLayout',0,'Factor',1,'Offset',0,'Min',0,'Max',255,'SgnComment',{{}},'SgnUnit',''),'MsgIdNumFormat',0,'MsgComment',{{''}}),'Version',1.2,'general',struct('isFromLib',1)),'GroupId',struct('Group',{{'RTICAN'}},'No',1,'Behavior',{{'NAMECHANGE'}},'BlockType',{{'SINK'}},'NameChangeFlag',0),'SFcnRTICANMessage',struct('MsgType','RX','MsgName',['RX Message'],'MsgIdFormat','STD','MsgId',100,'MsgLength',8,'NumSignals',1,'SampleTime',-1,'Signal',struct('SgnName',['RX signal'],'SgnStartBit',0,'SgnLength',8,'SgnType','standard','ModeValue',-1,'DataType',['unsigned int'],'ByteLayout',['little endian'],'SLDataType','SS_DOUBLE','Factor',1,'Offset',0),'StatusSelected','yes','TimeSelected','yes','DeltaTimeSelected','yes','BytePortSelected','no','MessageLengthSelected','no','EnablePortSelected','no','UserCoding',struct('Selected','no','InterfaceFile','UserDecodingFile','FcnName','UserDecodeFcn','InportSelected','no','InportWidth',1,'OutportSelected','no','OutportWidth',1),'TriggerPort',struct('Selected','no','TriggerType','rising'),'UseRXService','no','BoardType','DS4302','BoardNo',1,'ControllerNo',1,'SFcnPortType','Scalar'),'TLCFileName','rtican_rx_message')
      settings: AttributesFormatString=Group Id: RTICAN3\n
  Terminator{4..7,12..14} (7 alike) : Terminator
  wires:
  Speed Control PID Parameters/1 -> Terminator4/1  "PGainNumerator"
  Speed Control PID Parameters/2 -> Terminator5/1  "IGainNumerator"
  Speed Control PID Parameters/3 -> Terminator6/1  "DGainNumerator"
  Speed Control PID Parameters/4 -> Terminator7/1  "PIDDivisor"
  Speed Control PID Parameters/5 -> Terminator12/1
  Speed Control PID Parameters/6 -> Terminator13/1
  Speed Control PID Parameters/7 -> Terminator14/1

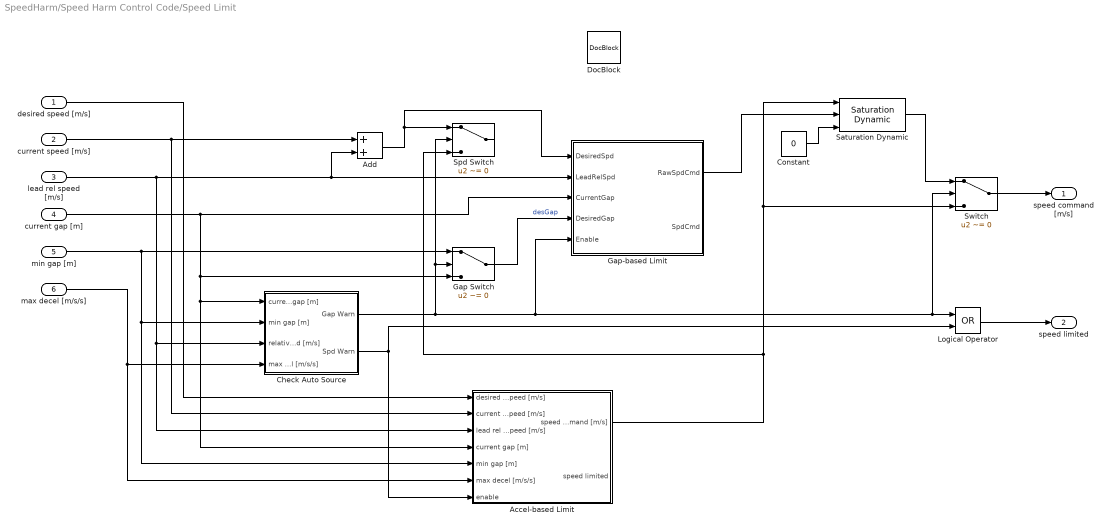
== system SpeedHarm/Speed Harm Control Code/Speed Limit ==
  desired speed [m/s] : Inport
  current speed [m/s] : Inport  Port=2
  lead rel speed [m/s] : Inport  Port=3
  current gap [m] : Inport  Port=4
  min gap [m] : Inport  Port=5
  max decel [m/s/s] : Inport  Port=6
  Accel-based Limit : Subsystem
  Add : Sum
  Check Auto Source : Subsystem
  Constant : Constant  Value=0
  DocBlock : simulink/Model-Wide Utilities/DocBlock  DocumentType=Text
  Gap Switch : Switch  Criteria=u2 ~= 0
  Gap-based Limit : Subsystem
  Logical Operator : Logic  Operator=OR  AllPortsSameDT=off  OutDataTypeStr='uint8'
  Saturation Dynamic : simulink/Discontinuities/Saturation Dynamic  OutMin=[]  OutMax=[]  OutDataTypeStr=Inherit: Same as second input  OutDataType=fixdt(1, 16)  OutScaling=2^-10  DoSatur=off
  Spd Switch : Switch  Criteria=u2 ~= 0
  Switch : Switch  Criteria=u2 ~= 0
  speed command [m/s] : Outport
  speed limited : Outport  Port=2
  wires:
  current gap [m]/1 -> Gap-based Limit/3(CurrentGap), Gap Switch/3, Accel-based Limit/4(current gap [m]), Check Auto Source/1(current gap [m])
  lead rel speed [m/s]/1 -> Gap-based Limit/2(LeadRelSpd), Add/2, Accel-based Limit/3(lead rel speed [m/s]), Check Auto Source/3(relative spd [m/s])
  Constant/1 -> Saturation Dynamic/3
  current speed [m/s]/1 -> Add/1, Accel-based Limit/2(current speed [m/s])
  desired speed [m/s]/1 -> Accel-based Limit/1(desired speed [m/s])
  min gap [m]/1 -> Gap Switch/1, Accel-based Limit/5(min gap [m]), Check Auto Source/2(min gap [m])
  Add/1 -> Spd Switch/1, Gap-based Limit/1(DesiredSpd)
  Gap-based Limit/1(RawSpdCmd) -> Saturation Dynamic/2
  Saturation Dynamic/1 -> Switch/1
  Check Auto Source/1(Gap Warn) -> Spd Switch/2, Gap Switch/2, Gap-based Limit/5(Enable), Logical Operator/1, Switch/2
  Gap Switch/1 -> Gap-based Limit/4(DesiredGap)  "desGap"
  max decel [m/s/s]/1 -> Accel-based Limit/6(max decel [m/s/s]), Check Auto Source/4(max decel [m/s/s])
  Check Auto Source/2(Spd Warn) -> Accel-based Limit/7(enable), Logical Operator/2
  Switch/1 -> speed command [m/s]/1
  Accel-based Limit/1(speed command [m/s]) -> Spd Switch/3, Saturation Dynamic/1, Switch/3
  Logical Operator/1 -> speed limited/1

== system SpeedHarm/Speed Harm Control Code/Speed Validation ==
  Value : Inport
  Abs : Abs
  Add : Sum
  DocBlock : simulink/Model-Wide Utilities/DocBlock  DocumentType=Text
      content=|
      | This block serves to limit the possible change per timestep for the
      | incoming signal.
  Memory : Memory  InheritSampleTime=on
  Saturation : Saturate  UpperLimit=1  LowerLimit=-1
  Subtract : Sum  Inputs=+-
  Switch : Switch  Criteria=u2 > Threshold  Threshold=1
  Filtered Value : Outport
  wires:
  Value/1 -> Subtract/1, Switch/3
  Memory/1 -> Add/1, Subtract/2
  Subtract/1 -> Abs/1, Saturation/1
  Switch/1 -> Memory/1, Filtered Value/1
  Abs/1 -> Switch/2
  Add/1 -> Switch/1
  Saturation/1 -> Add/2

== system SpeedHarm/Write CACC Data/Veh 1 Data Write ==
  DSRC Bus : Inport
  Action Port : ActionPort  ActionType=case
  Bus Selector : BusSelector  OutputSignals=signal1,signal2,signal3,signal4,signal5,signal6,signal7,signal8,signal9,signal10,signal11,signal12,signal13,signal14,signal15,signal16,signal17,signal18,signal19,signal20,signal21,signal22,signal23,signal24,signal25,signal26
  Data Store Write : DataStoreWrite  DataStoreName=BSMStoreSignal  DataStoreElements=BSMStoreSignal.Veh1BSM.grpID#BSMStoreSignal.Veh1BSM.grpSize#BSMStoreSignal.Veh1BSM.grpMode#BSMStoreSignal.Veh1BSM.grpManDes#BSMStoreSignal.Veh1BSM.grpManID#BSMStoreSignal.Veh1BSM.vehID#BSMStoreSignal.Veh1BSM.frntCutIn#BSMStoreSignal.Veh1BSM.vehGrpPos#BSMStoreSignal.Veh1BSM.vehFltMode#BSMStoreSignal.Veh1BSM.vehManDes#BSMStoreSignal.Veh1BSM.vehManID#BSMStoreSignal.Veh1BSM.distToPVeh_m#BSMStoreSignal.Veh1BSM.relSpdPVeh_m_s#BSMStoreSignal.Veh1BSM.distToLVeh_m#BSMStoreSignal.Veh1BSM.relSpdLVeh_m_s#BSMStoreSignal.Veh1BSM.desTGapPVeh_s#BSMStoreSignal.Veh1BSM.desTGapLVeh_s#BSMStoreSignal.Veh1BSM.estDisPVeh_m#BSMStoreSignal.Veh1BSM.estDisLVeh_m#BSMStoreSignal.Veh1BSM.desSpeed_m_s#BSMStoreSignal.Veh1BSM.desTrq_N_m#BSMStoreSignal.Veh1BSM.userDE1#BSMStoreSignal.Veh1BSM.userDE2#BSMStoreSignal.Veh1BSM.userDE3#BSMStoreSignal.Veh1BSM.userDE4#BSMStoreSignal.Veh1BSM.userDE5
  wires:
  Bus Selector/26 -> Data Store Write/26  "<signal26>"
  Bus Selector/25 -> Data Store Write/25  "<signal25>"
  Bus Selector/24 -> Data Store Write/24  "<signal24>"
  Bus Selector/23 -> Data Store Write/23  "<signal23>"
  Bus Selector/22 -> Data Store Write/22  "<signal22>"
  Bus Selector/21 -> Data Store Write/21  "<signal21>"
  Bus Selector/20 -> Data Store Write/20  "<signal20>"
  Bus Selector/19 -> Data Store Write/19  "<signal19>"
  Bus Selector/18 -> Data Store Write/18  "<signal18>"
  Bus Selector/17 -> Data Store Write/17  "<signal17>"
  Bus Selector/16 -> Data Store Write/16  "<signal16>"
  Bus Selector/15 -> Data Store Write/15  "<signal15>"
  Bus Selector/14 -> Data Store Write/14  "<signal14>"
  Bus Selector/13 -> Data Store Write/13  "<signal13>"
  Bus Selector/12 -> Data Store Write/12  "<signal12>"
  Bus Selector/11 -> Data Store Write/11  "<signal11>"
  Bus Selector/10 -> Data Store Write/10  "<signal10>"
  Bus Selector/9 -> Data Store Write/9  "<signal9>"
  Bus Selector/8 -> Data Store Write/8  "<signal8>"
  Bus Selector/7 -> Data Store Write/7  "<signal7>"
  Bus Selector/6 -> Data Store Write/6  "<signal6>"
  Bus Selector/5 -> Data Store Write/5  "<signal5>"
  Bus Selector/4 -> Data Store Write/4  "<signal4>"
  Bus Selector/3 -> Data Store Write/3  "<signal3>"
  Bus Selector/2 -> Data Store Write/2  "<signal2>"
  Bus Selector/1 -> Data Store Write/1  "<signal1>"
  DSRC Bus/1 -> Bus Selector/1

== system SpeedHarm/Write CACC Data/Veh 2 Data Write ==
  DSRC Bus : Inport
  Action Port : ActionPort  ActionType=case
  Bus Selector : BusSelector  OutputSignals=signal1,signal2,signal3,signal4,signal5,signal6,signal7,signal8,signal9,signal10,signal11,signal12,signal13,signal14,signal15,signal16,signal17,signal18,signal19,signal20,signal21,signal22,signal23,signal24,signal25,signal26
  Data Store Write : DataStoreWrite  DataStoreName=BSMStoreSignal  DataStoreElements=BSMStoreSignal.Veh2BSM.grpID#BSMStoreSignal.Veh2BSM.grpSize#BSMStoreSignal.Veh2BSM.grpMode#BSMStoreSignal.Veh2BSM.grpManDes#BSMStoreSignal.Veh2BSM.grpManID#BSMStoreSignal.Veh2BSM.vehID#BSMStoreSignal.Veh2BSM.frntCutIn#BSMStoreSignal.Veh2BSM.vehGrpPos#BSMStoreSignal.Veh2BSM.vehFltMode#BSMStoreSignal.Veh2BSM.vehManDes#BSMStoreSignal.Veh2BSM.vehManID#BSMStoreSignal.Veh2BSM.distToPVeh_m#BSMStoreSignal.Veh2BSM.relSpdPVeh_m_s#BSMStoreSignal.Veh2BSM.distToLVeh_m#BSMStoreSignal.Veh2BSM.relSpdLVeh_m_s#BSMStoreSignal.Veh2BSM.desTGapPVeh_s#BSMStoreSignal.Veh2BSM.desTGapLVeh_s#BSMStoreSignal.Veh2BSM.estDisPVeh_m#BSMStoreSignal.Veh2BSM.estDisLVeh_m#BSMStoreSignal.Veh2BSM.desSpeed_m_s#BSMStoreSignal.Veh2BSM.desTrq_N_m#BSMStoreSignal.Veh2BSM.userDE1#BSMStoreSignal.Veh2BSM.userDE2#BSMStoreSignal.Veh2BSM.userDE3#BSMStoreSignal.Veh2BSM.userDE4#BSMStoreSignal.Veh2BSM.userDE5
  wires:
  Bus Selector/26 -> Data Store Write/26  "<signal26>"
  Bus Selector/25 -> Data Store Write/25  "<signal25>"
  Bus Selector/24 -> Data Store Write/24  "<signal24>"
  Bus Selector/23 -> Data Store Write/23  "<signal23>"
  Bus Selector/22 -> Data Store Write/22  "<signal22>"
  Bus Selector/21 -> Data Store Write/21  "<signal21>"
  Bus Selector/20 -> Data Store Write/20  "<signal20>"
  Bus Selector/19 -> Data Store Write/19  "<signal19>"
  Bus Selector/18 -> Data Store Write/18  "<signal18>"
  Bus Selector/17 -> Data Store Write/17  "<signal17>"
  Bus Selector/16 -> Data Store Write/16  "<signal16>"
  Bus Selector/15 -> Data Store Write/15  "<signal15>"
  Bus Selector/14 -> Data Store Write/14  "<signal14>"
  Bus Selector/13 -> Data Store Write/13  "<signal13>"
  Bus Selector/12 -> Data Store Write/12  "<signal12>"
  Bus Selector/11 -> Data Store Write/11  "<signal11>"
  Bus Selector/10 -> Data Store Write/10  "<signal10>"
  Bus Selector/9 -> Data Store Write/9  "<signal9>"
  Bus Selector/8 -> Data Store Write/8  "<signal8>"
  Bus Selector/7 -> Data Store Write/7  "<signal7>"
  Bus Selector/6 -> Data Store Write/6  "<signal6>"
  Bus Selector/5 -> Data Store Write/5  "<signal5>"
  Bus Selector/4 -> Data Store Write/4  "<signal4>"
  Bus Selector/3 -> Data Store Write/3  "<signal3>"
  Bus Selector/2 -> Data Store Write/2  "<signal2>"
  Bus Selector/1 -> Data Store Write/1  "<signal1>"
  DSRC Bus/1 -> Bus Selector/1
